simulink model "SWC_FDC_type"  (R2021b)
settings: Solver=FixedStepDiscrete  StartTime=0.0  StopTime=10.0  FixedStep=0.001  RelTol=1e-3
values from neighbouring files (symbols this model uses):
  DID_VCUKey = uint16(0x0202)    [vcu_local_hdr.m]
  DID_XWD = uint16(513)    [vcu_local_hdr.m]
  DIDLen_DKCKey = uint16(8)    [vcu_local_hdr.m]
  DIDLen_DynoMode = uint16(1)    [vcu_local_hdr.m]
  DIDLen_LFLowPresThre = uint16(1)    [vcu_local_hdr.m]
  DIDLen_LFSensorID = uint16(4)    [vcu_local_hdr.m]
  DIDLen_LRLowPresThre = uint16(1)    [vcu_local_hdr.m]
  DIDLen_LRSensorID = uint16(4)    [vcu_local_hdr.m]
  DIDLen_RFLowPresThre = uint16(1)    [vcu_local_hdr.m]
  DIDLen_RFSensorID = uint16(4)    [vcu_local_hdr.m]
  DIDLen_RRLowPresThre = uint16(1)    [vcu_local_hdr.m]
  DIDLen_RRSensorID = uint16(4)    [vcu_local_hdr.m]
  DIDLen_SensorMode = uint16(1)    [vcu_local_hdr.m]
  DIDLen_TPMSLearnSta = uint16(1)    [vcu_local_hdr.m]
  DIDLen_WhlPres = uint16(4)    [vcu_local_hdr.m]
  DIDLen_WhlSensorBattSta = uint16(1)    [vcu_local_hdr.m]
  DIDLen_WhlTmp = uint16(4)    [vcu_local_hdr.m]
  DIDLen_XWDMode = uint16(1)    [vcu_local_hdr.m]
  DIDNum_DKCKey = uint16(0x0202)    [vcu_local_hdr.m]
  DIDNum_DynoMode = uint16(0x0203)    [vcu_local_hdr.m]
  DIDNum_LFLowPresThre = uint16(0x0B08)    [vcu_local_hdr.m]
  DIDNum_LFSensorID = uint16(0x0B01)    [vcu_local_hdr.m]
  DIDNum_LRLowPresThre = uint16(0x0B0A)    [vcu_local_hdr.m]
  DIDNum_LRSensorID = uint16(0x0B03)    [vcu_local_hdr.m]
  DIDNum_RFLowPresThre = uint16(0x0B09)    [vcu_local_hdr.m]
  DIDNum_RFSensorID = uint16(0x0B02)    [vcu_local_hdr.m]
  DIDNum_RRLowPresThre = uint16(0x0B0B)    [vcu_local_hdr.m]
  DIDNum_RRSensorID = uint16(0x0B04)    [vcu_local_hdr.m]
  DIDNum_SensorMode = uint16(0x0B0C)    [vcu_local_hdr.m]
  DIDNum_TPMSLearnSta = uint16(0x0B0D)    [vcu_local_hdr.m]
  DIDNum_WhlPres = uint16(0x0B05)    [vcu_local_hdr.m]
  DIDNum_WhlSensorBattSta = uint16(0x0B07)    [vcu_local_hdr.m]
  DIDNum_WhlTmp = uint16(0x0B06)    [vcu_local_hdr.m]
  DIDNum_XWDMode = uint16(0x0201)    [vcu_local_hdr.m]
  DIDVCUKeyLength = uint16(8)    [vcu_local_hdr.m]
  ENUM_DRIVETRAIN_AWD = uint8(  2  )    [vcu_local_hdr.m]
  ENUM_DRIVETRAIN_FWD = uint8(  1  )    [vcu_local_hdr.m]
  ENUM_DRIVETRAIN_RWD = uint8(  0  )    [vcu_local_hdr.m]
  ENUM_TPMSLearnStatus_LEARNED = uint8(  1  )    [vcu_local_hdr.m]
  ENUM_TPMSLearnStatus_LEARNFAIL = uint8(  2  )    [vcu_local_hdr.m]
  ENUM_TPMSLearnStatus_NOTLEARN = uint8(  0  )    [vcu_local_hdr.m]
  ENUM_TPMSSTA_FAT = uint8(  8  )    [vcu_local_hdr.m]
  ENUM_TPMSSTA_LOWBATTERY = uint8(  2  )    [vcu_local_hdr.m]
  FALSE = boolean( 0 )    [vcu_local_hdr.m]
  ONE_INT = uint8(1)    [vcu_local_hdr.m]
  P_boolean = 0.0    [APPTypes.sldd]
  TRUE = boolean( 1 )    [vcu_local_hdr.m]
  ZERO_FLOAT = single(0)    [vcu_local_hdr.m]
  ZERO_INT = uint8(0)    [vcu_local_hdr.m]
undefined symbols (not defined in the file or in its folder): f32_ApsOutVehSpdSig, KHAL_DKCDecryptEnable_flg_ovrdflg, KHAL_DKCDecryptEnable_flg_ovrdval, KHAL_RandomNumberY1_enum, KHAL_RandomNumberY2_enum, KHAL_RandomNumberY_ovrdflg, KHAL_TPMSRESBUTT_flg_ovrdflg, KHAL_TPMSRESBUTT_flg_ovrdval, R_DIDWriteCDD_CSOP_DIDSet_DKCKey, R_DIDWriteCDD_CSOP_DIDSet_DynoMode, R_DIDWriteCDD_CSOP_DIDSet_LFLowPresThre, R_DIDWriteCDD_CSOP_DIDSet_LFSensorID, R_DIDWriteCDD_CSOP_DIDSet_LRLowPresThre, R_DIDWriteCDD_CSOP_DIDSet_LRSensorID, R_DIDWriteCDD_CSOP_DIDSet_RFLowPresThre, R_DIDWriteCDD_CSOP_DIDSet_RFSensorID, R_DIDWriteCDD_CSOP_DIDSet_RRLowPresThre, R_DIDWriteCDD_CSOP_DIDSet_RRSensorID, R_DIDWriteCDD_CSOP_DIDSet_SensorMode, R_DIDWriteCDD_CSOP_DIDSet_TPMSLearnSta, R_DIDWriteCDD_CSOP_DIDSet_WhlPres, R_DIDWriteCDD_CSOP_DIDSet_WhlSensorBattSta, R_DIDWriteCDD_CSOP_DIDSet_WhlTmp, R_DIDWriteCDD_CSOP_DIDSet_XWDMode, R_E2E_CAN3_VCU1_CSOP_Write_CAN3_VCU1, R_E2E_CAN4_VCU1_CSOP_Write_CAN4_VCU1, R_FDCCDD_Inner_CSOP_FDC_AppCallSleep, R_HALIN_IMU_CSOP_IMUSetSta, R_HALINCDD_CSOP_PAS_Handler, R_HALINCDD_CSOP_UDS_Main, R_HALOUT_APS_CSOP_ApsOutput, R_HALOUTCDD_CSOP_AppNmStateReq, R_HALOUTCDD_CSOP_IVIReset, R_HALOUTCDD_CSOP_SetAcoreRebootCmdACK, R_HALOUTCDD_CSOP_SetSysPwrStat, R_HALOUTCDD_CSOP_SleepRequest, R_NVMReadCDD_Inner_NVM_ReadOperation, R_NVMWriteCDD_Inner_NVM_WriteOperation, R_UDSCDD_CSOP_DdmRestartOperationCycle, R_WDGCDD_CSOP_Call_Watchdog, R_WDGCDD_CSOP_Call_WDG_AppEnd, R_WDGCDD_CSOP_Call_WDG_AppStart, u16_DIDLen_DKCKey, u16_DIDLen_DynoMode, u16_DIDLen_LFLowPresThre, u16_DIDLen_LFSensorID, u16_DIDLen_LRLowPresThre, u16_DIDLen_LRSensorID, u16_DIDLen_RFLowPresThre, u16_DIDLen_RFSensorID, u16_DIDLen_RRLowPresThre, u16_DIDLen_RRSensorID, u16_DIDLen_SensorMode, u16_DIDLen_TPMSLearnSta, u16_DIDLen_WhlPres, u16_DIDLen_WhlSensorBattSta, u16_DIDLen_WhlTmp, u16_DIDLen_XWDMode, u16_DIDNum_DKCKey, u16_DIDNum_DynoMode ... (+42)
libraries: simulink x215, FVT_lib x137, hcu_lib x12, hdlsllib x9, app x1, halin x1, halout x1, inp x1, outp x1
(part 4 of 11)

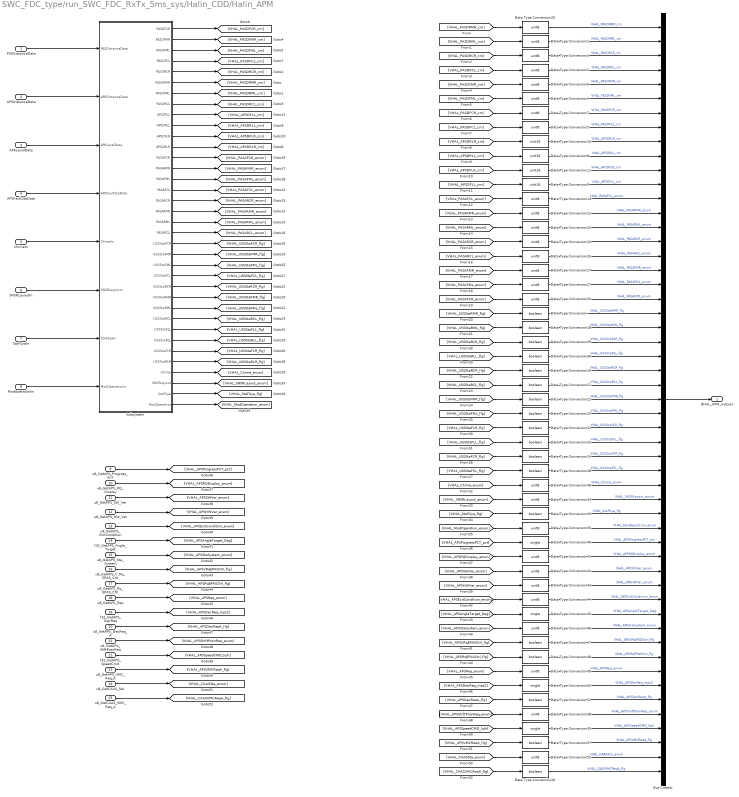
== system SWC_FDC_type/run_SWC_FDC_RxTx_5ms_sys/Halin_CDD/Halin_APM ==
  PASDistanceData : Inport
  APSDistanceData : Inport  Port=2
  APSLevelData : Inport  Port=3
  APSFaultStaData : Inport  Port=4
  ChimeIn : Inport  Port=5
  SNSRLayoutIn : Inport  Port=6
  StaFSyaIn : Inport  Port=7
  ModOperationIn : Inport  Port=8
  u8_GetAPS_Progress_PCT : Inport  Port=9
  u8_GetAPS_RQ_Display : Inport  Port=10
  u8_GetAPS_SW_Ver : Inport  Port=11
  u8_GetAPS_HW_Ver : Inport  Port=12
  u8_GetAPS_ExitCondition : Inport  Port=13
  f32_GetAPS_Angle_Target : Inport  Port=14
  u8_GetAPS_Sta_System : Inport  Port=15
  u8_GetAPS_V_Rq_EPAS_Ctrl : Inport  Port=16
  u8_GetAPS_Rq_EPAS_Ctrl : Inport  Port=17
  u8_GetAPS_Req : Inport  Port=18
  f32_GetAPS_DecReq : Inport  Port=19
  u8_GetAPS_DecReq_A : Inport  Port=20
  f32_GetAPS_SpeedCmd : Inport  Port=21
  u8_GetAPS_ShftPosnReq : Inport  Port=22
  u8_GetAPS_VMC_Req_A : Inport  Port=23
  u8_GetCAAS_Sta : Inport  Port=24
  u8_GetCAAS_VMC_Req_A : Inport  Port=25
  Bus Creator : BusCreator  Inputs=53
  Data Type Conversion{,16,18..19,21..24,28..33,37,47..48,51} (18 alike) : DataTypeConversion  OutDataTypeStr=boolean
  Data Type Conversion{1..7,12..15,17,20,25..27,34..36,38,41..44,46,49,52} (27 alike) : DataTypeConversion  OutDataTypeStr=uint8
  Data Type Conversion{8..11} (4 alike) : DataTypeConversion  OutDataTypeStr=uint16
  Data Type Conversion{39..40,45,50} (4 alike) : DataTypeConversion  OutDataTypeStr=single
  Subsystem : Subsystem
  BHAL_APM_outputs : Outport
  wires:
  [VHAL_USSStaRMR_flg] -> Data Type Conversion/1
  Data Type Conversion4/1 -> Bus Creator/6  "VHAL_PASDFML_cm"
  Subsystem/11(APSDFLR) -> [VHAL_APSDFLR_cm]
  [VHAL_PASARCL_enum] -> Data Type Conversion26/1
  Subsystem/36(ModOperation) -> [VHAL_ModOperation_enum]
  Bus Creator/1 -> BHAL_APM_outputs/1
  [VHAL_PASDRCR_cm] -> Data Type Conversion3/1
  [VHAL_PASDRML_cm] -> Data Type Conversion1/1
  Data Type Conversion15/1 -> Bus Creator/15  "VHAL_PASARML_enum"
  [VHAL_USSStaFCR_flg] -> Data Type Conversion24/1
  [VHAL_SNSRLayout_enum] -> Data Type Conversion34/1
  Subsystem/12(APSDRLR) -> [VHAL_APSDRLR_cm]
  Data Type Conversion3/1 -> Bus Creator/3  "VHAL_PASDRCR_cm"
  [VHAL_APSDRLR_cm] -> Data Type Conversion10/1
  Data Type Conversion12/1 -> Bus Creator/14  "VHAL_PASARMR_enum"
  Data Type Conversion33/1 -> Bus Creator/35  "VHAL_StaFSya_flg"
  [VHAL_PASARCR_enum] -> Data Type Conversion13/1
  Subsystem/9(APSDFLL) -> [VHAL_APSDFLL_cm]
  [VHAL_StaFSya_flg] -> Data Type Conversion33/1
  [VHAL_USSStaRLL_flg] -> Data Type Conversion30/1
  Subsystem/4(PASDFCL) -> [VHAL_PASDFCL_cm]
  Subsystem/35(StaFSya) -> [VHAL_StaFSya_flg]
  Subsystem/20(PASARCL) -> [VHAL_PASARCL_enum]
  [VHAL_PASDFML_cm] -> Data Type Conversion4/1
  [VHAL_PASDRMR_cm] -> Data Type Conversion20/1
  Subsystem/16(PASAFCL) -> [VHAL_PASAFCL_enum]
  [VHAL_USSStaFCL_flg] -> Data Type Conversion28/1
  Subsystem/18(PASARMR) -> [VHAL_PASARMR_enum]
  Data Type Conversion13/1 -> Bus Creator/16  "VHAL_PASARCR_enum"
  [VHAL_PASARML_enum] -> Data Type Conversion15/1
  [VHAL_APSDFLL_cm] -> Data Type Conversion9/1
  Subsystem/15(PASAFML) -> [VHAL_PASAFML_enum]
  [VHAL_USSStaFLL_flg] -> Data Type Conversion32/1
  Subsystem/8(PASDRCL) -> [VHAL_PASDRCL_cm]
  Subsystem/27(USSStaRML) -> [VHAL_USSStaRML_flg]
  Data Type Conversion6/1 -> Bus Creator/5  "VHAL_PASDFMR_cm"
  [VHAL_PASAFMR_enum] -> Data Type Conversion17/1
  Data Type Conversion28/1 -> Bus Creator/32  "VHAL_USSStaFCL_flg"
  Subsystem/3(PASDFML) -> [VHAL_PASDFML_cm]
  Data Type Conversion9/1 -> Bus Creator/12  "VHAL_APSDFLL_cm"
  Subsystem/24(USSStaFCL) -> [VHAL_USSStaFCL_flg]
  [VHAL_PASAFCL_enum] -> Data Type Conversion14/1
  [VHAL_USSStaFLR_flg] -> Data Type Conversion31/1
  Subsystem/34(SNSRLayout) -> [VHAL_SNSRLayout_enum]
  Subsystem/29(USSStaFLL) -> [VHAL_USSStaFLL_flg]
  Subsystem/21(USSStaFCR) -> [VHAL_USSStaFCR_flg]
  [VHAL_PASDRCL_cm] -> Data Type Conversion2/1
  Data Type Conversion14/1 -> Bus Creator/13  "VHAL_PASAFCL_enum"
  Subsystem/1(PASDFCR) -> [VHAL_PASDFCR_cm]
  Data Type Conversion7/1 -> Bus Creator/7  "VHAL_PASDFCR_cm"
  Subsystem/2(PASDFMR) -> [VHAL_PASDFMR_cm]
  Subsystem/30(USSStaRLL) -> [VHAL_USSStaRLL_flg]
  Data Type Conversion17/1 -> Bus Creator/18  "VHAL_PASAFMR_enum"
  [VHAL_PASARMR_enum] -> Data Type Conversion12/1
  Data Type Conversion32/1 -> Bus Creator/30  "VHAL_USSStaFLL_flg"
  Subsystem/7(PASDRML) -> [VHAL_PASDRML_cm]
  Subsystem/26(USSStaRMR) -> [VHAL_USSStaRMR_flg]
  Data Type Conversion20/1 -> Bus Creator/1  "VHAL_PASDRMR_cm"
  [VHAL_USSStaRCL_flg] -> Data Type Conversion21/1
  Subsystem/10(APSDRLL) -> [VHAL_APSDRLL_cm]
  Data Type Conversion34/1 -> Bus Creator/34  "VHAL_SNSRLayout_enum"
  [VHAL_Chime_enum] -> Data Type Conversion36/1
  Data Type Conversion18/1 -> Bus Creator/22  "VHAL_USSStaRML_flg"
  [VHAL_PASDFMR_cm] -> Data Type Conversion6/1
  Data Type Conversion31/1 -> Bus Creator/29  "VHAL_USSStaFLR_flg"
  Data Type Conversion10/1 -> Bus Creator/9  "VHAL_APSDRLR_cm"
  Data Type Conversion35/1 -> Bus Creator/36  "VHAL_ModOperation_enum"
  Subsystem/31(USSStaFLR) -> [VHAL_USSStaFLR_flg]
  Data Type Conversion8/1 -> Bus Creator/10  "VHAL_APSDRLL_cm"
  [VHAL_USSStaRML_flg] -> Data Type Conversion18/1
  Subsystem/19(PASARML) -> [VHAL_PASARML_enum]
  [VHAL_USSStaFMR_flg] -> Data Type Conversion22/1
  Subsystem/22(USSStaFMR) -> [VHAL_USSStaFMR_flg]
  Data Type Conversion25/1 -> Bus Creator/20  "VHAL_PASAFCR_enum"
  Subsystem/33(Chime) -> [VHAL_Chime_enum]
  Data Type Conversion11/1 -> Bus Creator/11  "VHAL_APSDFLR_cm"
  Data Type Conversion36/1 -> Bus Creator/33  "VHAL_Chime_enum"
  [VHAL_APSDFLR_cm] -> Data Type Conversion11/1
  Subsystem/13(PASAFCR) -> [VHAL_PASAFCR_enum]
  [VHAL_PASDFCL_cm] -> Data Type Conversion5/1
  Data Type Conversion/1 -> Bus Creator/21  "VHAL_USSStaRMR_flg"
  Data Type Conversion2/1 -> Bus Creator/4  "VHAL_PASDRCL_cm"
  [VHAL_USSStaFML_flg] -> Data Type Conversion23/1
  Data Type Conversion1/1 -> Bus Creator/2  "VHAL_PASDRML_cm"
  [VHAL_USSStaRCR_flg] -> Data Type Conversion19/1
  Subsystem/25(USSStaRCR) -> [VHAL_USSStaRCR_flg]
  Subsystem/28(USSStaRCL) -> [VHAL_USSStaRCL_flg]
  [VHAL_ModOperation_enum] -> Data Type Conversion35/1
  Data Type Conversion19/1 -> Bus Creator/25  "VHAL_USSStaRCR_flg"
  Subsystem/5(PASDRCR) -> [VHAL_PASDRCR_cm]
  Data Type Conversion26/1 -> Bus Creator/17  "VHAL_PASARCL_enum"
  Data Type Conversion27/1 -> Bus Creator/19  "VHAL_PASAFML_enum"
  Subsystem/23(USSStaFML) -> [VHAL_USSStaFML_flg]
  Subsystem/17(PASARCR) -> [VHAL_PASARCR_enum]
  [VHAL_APSDRLL_cm] -> Data Type Conversion8/1
  Subsystem/6(PASDRMR) -> [VHAL_PASDRMR_cm]
  Data Type Conversion21/1 -> Bus Creator/26  "VHAL_USSStaRCL_flg"
  Data Type Conversion24/1 -> Bus Creator/31  "VHAL_USSStaFCR_flg"
  Data Type Conversion23/1 -> Bus Creator/28  "VHAL_USSStaFML_flg"
  Data Type Conversion5/1 -> Bus Creator/8  "VHAL_PASDFCL_cm"
  [VHAL_PASAFCR_enum] -> Data Type Conversion25/1
  [VHAL_PASDFCR_cm] -> Data Type Conversion7/1
  Data Type Conversion29/1 -> Bus Creator/23  "VHAL_USSStaRLR_flg"
  [VHAL_USSStaRLR_flg] -> Data Type Conversion29/1
  Subsystem/14(PASAFMR) -> [VHAL_PASAFMR_enum]
  Data Type Conversion30/1 -> Bus Creator/24  "VHAL_USSStaRLL_flg"
  Subsystem/32(USSStaRLR) -> [VHAL_USSStaRLR_flg]
  [VHAL_PASAFML_enum] -> Data Type Conversion27/1
  Data Type Conversion22/1 -> Bus Creator/27  "VHAL_USSStaFMR_flg"
  APSDistanceData/1 -> Subsystem/2(APSDistanceData)
  APSFaultStaData/1 -> Subsystem/4(APSFaultStaData)
  APSLevelData/1 -> Subsystem/3(APSLevelData)
  ChimeIn/1 -> Subsystem/5(ChimeIn)
  SNSRLayoutIn/1 -> Subsystem/6(SNSRLayoutIn)
  StaFSyaIn/1 -> Subsystem/7(StaFSyaIn)
  ModOperationIn/1 -> Subsystem/8(ModOperationIn)
  PASDistanceData/1 -> Subsystem/1(PASDistanceData)
  u8_GetAPS_HW_Ver/1 -> [VHAL_APSHWVer_enum]
  u8_GetAPS_Progress_PCT/1 -> [VHAL_APSProgressPCT_pct]
  u8_GetAPS_Req/1 -> [VHAL_APSReq_enum]
  u8_GetAPS_Sta_System/1 -> [VHAL_APSStaSystem_enum]
  u8_GetAPS_SW_Ver/1 -> [VHAL_APSSWVer_enum]
  u8_GetAPS_V_Rq_EPAS_Ctrl/1 -> [VHAL_APSVRqEPASCtrl_flg]
  u8_GetAPS_ExitCondition/1 -> [VHAL_APSExitCondition_enum]
  u8_GetCAAS_Sta/1 -> [VHAL_CAASSta_enum]
  u8_GetAPS_VMC_Req_A/1 -> [VHAL_APSVMCReqA_flg]
  f32_GetAPS_SpeedCmd/1 -> [VHAL_APSSpeedCMD_kph]
  u8_GetAPS_Rq_EPAS_Ctrl/1 -> [VHAL_APSRqEPASCtrl_flg]
  u8_GetAPS_ShftPosnReq/1 -> [VHAL_APSShiftPosnReq_enum]
  u8_GetAPS_DecReq_A/1 -> [VHAL_APSDecReqA_flg]
  f32_GetAPS_Angle_Target/1 -> [VHAL_APSAngleTarget_Deg]
  u8_GetAPS_RQ_Display/1 -> [VHAL_APSRQDisplay_enum]
  f32_GetAPS_DecReq/1 -> [VHAL_APSDecReq_mps2]
  u8_GetCAAS_VMC_Req_A/1 -> [VHAL_CAASVMCReqA_flg]
  Data Type Conversion47/1 -> Bus Creator/44  "VHAL_APSVRqEPASCtrl_flg"
  Data Type Conversion50/1 -> Bus Creator/47  "VHAL_APSDecReq_mps2"
  Data Type Conversion39/1 -> Bus Creator/50  "VHAL_APSSpeedCMD_kph"
  Data Type Conversion43/1 -> Bus Creator/40  "VHAL_APSHWVer_enum"
  Data Type Conversion38/1 -> Bus Creator/49  "VHAL_APSShiftPosnReq_enum"
  Data Type Conversion42/1 -> Bus Creator/39  "VHAL_APSSWVer_enum"
  [VHAL_APSVRqEPASCtrl_flg] -> Data Type Conversion47/1
  Data Type Conversion51/1 -> Bus Creator/48  "VHAL_APSDecReqA_flg"
  Data Type Conversion46/1 -> Bus Creator/43  "VHAL_APSStaSystem_enum"
  Data Type Conversion44/1 -> Bus Creator/41  "VHAL_APSExitCondition_enum"
  [VHAL_APSVMCReqA_flg] -> Data Type Conversion37/1
  [VHAL_APSReq_enum] -> Data Type Conversion49/1
  [VHAL_APSSpeedCMD_kph] -> Data Type Conversion39/1
  Data Type Conversion48/1 -> Bus Creator/45  "VHAL_APSRqEPASCtrl_flg"
  [VHAL_APSShiftPosnReq_enum] -> Data Type Conversion38/1
  Data Type Conversion52/1 -> Bus Creator/52  "VHAL_CAASSta_enum"
  Data Type Conversion45/1 -> Bus Creator/42  "VHAL_APSAngleTarget_Deg"
  Data Type Conversion49/1 -> Bus Creator/46  "VHAL_APSReq_enum"
  [VHAL_CAASSta_enum] -> Data Type Conversion52/1
  [VHAL_APSRqEPASCtrl_flg] -> Data Type Conversion48/1
  [VHAL_APSStaSystem_enum] -> Data Type Conversion46/1
  Data Type Conversion40/1 -> Bus Creator/37  "VHAL_APSProgressPCT_pct"
  [VHAL_APSExitCondition_enum] -> Data Type Conversion44/1
  [VHAL_APSSWVer_enum] -> Data Type Conversion42/1
  [VHAL_APSHWVer_enum] -> Data Type Conversion43/1
  [VHAL_APSAngleTarget_Deg] -> Data Type Conversion45/1
  [VHAL_APSDecReq_mps2] -> Data Type Conversion50/1
  [VHAL_APSProgressPCT_pct] -> Data Type Conversion40/1
  [VHAL_APSDecReqA_flg] -> Data Type Conversion51/1
  [VHAL_APSRQDisplay_enum] -> Data Type Conversion41/1
  Data Type Conversion41/1 -> Bus Creator/38  "VHAL_APSRQDisplay_enum"
  Data Type Conversion37/1 -> Bus Creator/51  "VHAL_APSVMCReqA_flg"
  [VHAL_CAASVMCReqA_flg] -> Data Type Conversion16/1
  Data Type Conversion16/1 -> Bus Creator/53  "VHAL_CAASVMCReqA_flg"

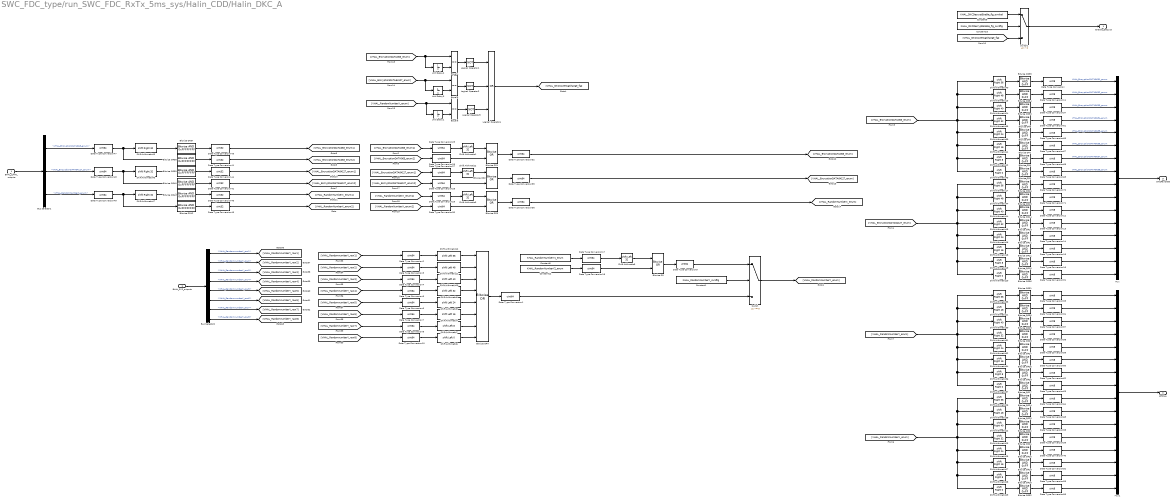
== system SWC_FDC_type/run_SWC_FDC_RxTx_5ms_sys/Halin_CDD/Halin_DKC_A ==
  BHAL_CAN4_outputs : Inport
  BHAL_SYS_outputs : Inport  Port=2
  Bitwise OR{,1..3} (4 alike) : simulink/Logic and Bit Operations/Bitwise Operator  logicop=OR  UseBitMask=off  NumInputPorts=2  BitMask=bin2dec('11011001')  BitMaskRealWorld=Stored Integer
  Bitwise OR{5..36} (32 alike) : simulink/Logic and Bit Operations/Bitwise Operator  logicop=AND  UseBitMask=on  BitMask=0xFF  BitMaskRealWorld=Stored Integer
  Bitwise OR{37..42} (6 alike) : simulink/Logic and Bit Operations/Bitwise Operator  logicop=AND  UseBitMask=on  BitMask=0xFFFFFFFF  BitMaskRealWorld=Stored Integer
  Bitwise OR4 : simulink/Logic and Bit Operations/Bitwise Operator  logicop=OR  UseBitMask=off  NumInputPorts=8  BitMask=bin2dec('11011001')  BitMaskRealWorld=Stored Integer
  Bus Selector1 : BusSelector  OutputSignals=VHAL_EncryptionDATA063_enum,VHAL_EncryptionDATA64127_enum,VHAL_RandomNumberX_enum
  Bus Selector2 : BusSelector  OutputSignals=VHAL_RandomnumberY_raw1,VHAL_RandomnumberY_raw2,VHAL_RandomnumberY_raw3,VHAL_RandomnumberY_raw4,VHAL_RandomnumberY_raw5,VHAL_RandomnumberY_raw6,VHAL_RandomnumberY_raw7,VHAL_RandomnumberY_raw8
  Constant1 : Constant  Value=KHAL_RandomNumberY_ovrdflg  OutDataTypeStr=uint64
  Constant10 : Constant  Value=KHAL_DKCDecryptEnable_flg_ovrdflg
  Constant12 : Constant  Value=KHAL_RandomNumberY2_enum  OutDataTypeStr=uint64
  Constant5 : Constant  Value=KHAL_RandomNumberY1_enum  OutDataTypeStr=uint64
  Constant9 : Constant  Value=KHAL_DKCDecryptEnable_flg_ovrdval
  Data Type Conversion{,11..16,31,33..34,37..40,52,55..71} (32 alike) : DataTypeConversion  OutDataTypeStr=uint8
  Data Type Conversion{1..10,17..18,25..30,32,35..36,47..49} (24 alike) : DataTypeConversion  OutDataTypeStr=uint64
  Data Type Conversion{41..46} (6 alike) : DataTypeConversion  OutDataTypeStr=uint32
  Equal4 : RelationalOperator  Operator===  OutDataTypeStr=boolean  RndMeth=Simplest
  Equal5 : RelationalOperator  Operator===  OutDataTypeStr=boolean  RndMeth=Simplest
  Equal6 : RelationalOperator  Operator===  OutDataTypeStr=boolean  RndMeth=Simplest
  Logical Operator1 : Logic  Operator=NOT  AllPortsSameDT=off  OutDataTypeStr=boolean
  Logical Operator2 : Logic  Operator=NOT  AllPortsSameDT=off  OutDataTypeStr=boolean
  Logical Operator3 : Logic  Operator=NOT  AllPortsSameDT=off  OutDataTypeStr=boolean
  Logical Operator4 : Logic  Operator=OR  Inputs=3  AllPortsSameDT=off  OutDataTypeStr=boolean
  Mux : Mux  Inputs=16
  Mux1 : Mux  Inputs=16
  Shift Arithmetic{1..3,5,9} (5 alike) : ArithShift  BitShiftNumber=32  BitShiftDirection=Left
  Shift Arithmetic10 : ArithShift  BitShiftNumber=40  BitShiftDirection=Left
  Shift Arithmetic11 : ArithShift  BitShiftNumber=48  BitShiftDirection=Left
  Shift Arithmetic12 : ArithShift  BitShiftNumber=56  BitShiftDirection=Left
  Shift Arithmetic{13,21,38,44} (4 alike) : ArithShift  BitShiftNumber=48  BitShiftDirection=Right
  Shift Arithmetic{14,22,24,30} (4 alike) : ArithShift  BitShiftNumber=40  BitShiftDirection=Right
  Shift Arithmetic{15,23,31,35,45..47} (7 alike) : ArithShift  BitShiftNumber=32  BitShiftDirection=Right
  Shift Arithmetic{16,25,32,39} (4 alike) : ArithShift  BitShiftNumber=24  BitShiftDirection=Right
  Shift Arithmetic{17,26,33,40} (4 alike) : ArithShift  BitShiftNumber=56  BitShiftDirection=Right
  Shift Arithmetic{18,27,34,41} (4 alike) : ArithShift  BitShiftNumber=16  BitShiftDirection=Right
  Shift Arithmetic{19,28,36,42} (4 alike) : ArithShift  BitShiftNumber=8  BitShiftDirection=Right
  Shift Arithmetic{20,29,37,43} (4 alike) : ArithShift  BitShiftDirection=Right
  Shift Arithmetic4 : ArithShift  BitShiftNumber=16  BitShiftDirection=Left
  Shift Arithmetic6 : ArithShift  BitShiftDirection=Left
  Shift Arithmetic7 : ArithShift  BitShiftNumber=8  BitShiftDirection=Left
  Shift Arithmetic8 : ArithShift  BitShiftNumber=24  BitShiftDirection=Left
  Switch : Switch  Criteria=u2 ~= 0
  Switch1 : Switch  Criteria=u2 > Threshold
  Unit Delay1 : UnitDelay  SampleTime=-1  HasFrameUpgradeWarning=on
  Unit Delay2 : UnitDelay  SampleTime=-1  HasFrameUpgradeWarning=on
  Unit Delay3 : UnitDelay  SampleTime=-1  HasFrameUpgradeWarning=on
  Enable_Decrypt : Outport
  AESKey : Outport  Port=2
  DKCRawData : Outport  Port=3
  wires:
  Data Type Conversion8/1 -> Shift Arithmetic7/1
  Bitwise OR5/1 -> Data Type Conversion69/1
  [VHAL_RandomNumberX_enum] -> Shift Arithmetic38/1, Shift Arithmetic26/1, Shift Arithmetic22/1, Shift Arithmetic25/1, Shift Arithmetic27/1, Shift Arithmetic29/1, Shift Arithmetic28/1, Shift Arithmetic23/1
  Shift Arithmetic17/1 -> Bitwise OR16/1
  Data Type Conversion52/1 -> Mux1/14
  Bitwise OR35/1 -> Data Type Conversion/1
  Shift Arithmetic13/1 -> Bitwise OR34/1
  Data Type Conversion42/1 -> [VHAL_EncryptionDATA64127_enum2]
  Bitwise OR/1 -> Data Type Conversion9/1
  [VHAL_EncryptionDATA64127_enum] -> Shift Arithmetic15/1, Shift Arithmetic19/1, Shift Arithmetic20/1, Shift Arithmetic18/1, Shift Arithmetic16/1, Shift Arithmetic14/1, Shift Arithmetic17/1, Shift Arithmetic44/1
  [VHAL_RandomnumberY_raw5] -> Data Type Conversion6/1
  Shift Arithmetic7/1 -> Bitwise OR4/7
  [VHAL_RandomnumberY_raw4] -> Data Type Conversion5/1
  [VHAL_RandomNumberX_enum] -> Equal6/1, Unit Delay1/1
  [VHAL_EncryptionDATA063_enum] -> Shift Arithmetic13/1, Shift Arithmetic40/1, Shift Arithmetic24/1, Shift Arithmetic39/1, Shift Arithmetic41/1, Shift Arithmetic43/1, Shift Arithmetic42/1, Shift Arithmetic35/1
  Bus Selector2/3 -> [VHAL_RandomnumberY_raw3]  "<VHAL_RandomnumberY_raw3>"
  Bitwise OR15/1 -> Data Type Conversion71/1
  Bus Selector2/2 -> [VHAL_RandomnumberY_raw2]  "<VHAL_RandomnumberY_raw2>"
  [VHAL_RandomnumberY_raw1] -> Data Type Conversion2/1
  Data Type Conversion69/1 -> Mux/8  "VHAL_EncryptionDATA0638_enum"
  Data Type Conversion37/1 -> Mux/3  "VHAL_EncryptionDATA0633_enum"
  Data Type Conversion5/1 -> Shift Arithmetic9/1
  Bitwise OR8/1 -> Data Type Conversion66/1
  Bitwise OR14/1 -> Data Type Conversion12/1
  Bus Selector2/1 -> [VHAL_RandomnumberY_raw1]  "<VHAL_RandomnumberY_raw1>"
  Bitwise OR17/1 -> Data Type Conversion63/1
  Data Type Conversion34/1 -> Mux1/2
  Bus Selector2/5 -> [VHAL_RandomnumberY_raw5]  "<VHAL_RandomnumberY_raw5>"
  Shift Arithmetic35/1 -> Bitwise OR9/1
  Data Type Conversion67/1 -> Mux/6  "VHAL_EncryptionDATA0636_enum"
  Bus Selector2/6 -> [VHAL_RandomnumberY_raw6]  "<VHAL_RandomnumberY_raw6>"
  Data Type Conversion9/1 -> Switch/1
  Data Type Conversion10/1 -> Shift Arithmetic6/1
  Data Type Conversion45/1 -> [VHAL_RandomNumberX_enum2]
  Data Type Conversion13/1 -> Mux/12
  Data Type Conversion1/1 -> Switch/3
  [VHAL_RandomnumberY_raw2] -> Data Type Conversion3/1
  BHAL_SYS_outputs/1 -> Bus Selector2/1
  Shift Arithmetic25/1 -> Bitwise OR20/1
  [VHAL_EncryptionDATA063_enum1] -> Data Type Conversion25/1
  Logical Operator3/1 -> Logical Operator4/3
  Shift Arithmetic6/1 -> Bitwise OR4/8
  Data Type Conversion70/1 -> Mux/9
  Data Type Conversion66/1 -> Mux/5  "VHAL_EncryptionDATA0635_enum"
  [VHAL_EncryptionDATA64127_enum] -> Equal5/1, Unit Delay3/1
  Data Type Conversion14/1 -> Mux/13
  Shift Arithmetic10/1 -> Bitwise OR4/3
  Data Type Conversion40/1 -> Mux1/13
  Unit Delay1/1 -> Equal6/2
  Data Type Conversion43/1 -> [VHAL_EncryptionDATA063_enum1]
  Unit Delay3/1 -> Equal5/2
  Bitwise OR31/1 -> Data Type Conversion33/1
  Shift Arithmetic12/1 -> Bitwise OR4/1
  [VHAL_RandomnumberY_raw3] -> Data Type Conversion4/1
  Shift Arithmetic28/1 -> Bitwise OR18/1
  Constant1/1 -> Switch/2
  Data Type Conversion7/1 -> Shift Arithmetic4/1
  Bitwise OR4/1 -> Data Type Conversion1/1
  Bitwise OR21/1 -> Data Type Conversion39/1
  Shift Arithmetic11/1 -> Bitwise OR4/2
  Data Type Conversion31/1 -> Mux/16
  Shift Arithmetic2/1 -> Bitwise OR2/1
  Data Type Conversion68/1 -> Mux/7  "VHAL_EncryptionDATA0637_enum"
  Data Type Conversion4/1 -> Shift Arithmetic10/1
  Bus Selector2/7 -> [VHAL_RandomnumberY_raw7]  "<VHAL_RandomnumberY_raw7>"
  Data Type Conversion12/1 -> Mux/11
  Data Type Conversion30/1 -> Bitwise OR3/2
  Data Type Conversion32/1 -> [VHAL_EncryptionDATA063_enum]
  [VHAL_RandomNumberY_enum] -> Shift Arithmetic31/1, Shift Arithmetic36/1, Shift Arithmetic37/1, Shift Arithmetic34/1, Shift Arithmetic32/1, Shift Arithmetic30/1, Shift Arithmetic33/1, Shift Arithmetic21/1
  Shift Arithmetic14/1 -> Bitwise OR14/1
  Data Type Conversion55/1 -> Mux1/15
  Shift Arithmetic33/1 -> Bitwise OR31/1
  Data Type Conversion59/1 -> Mux1/5
  Shift Arithmetic21/1 -> Bitwise OR30/1
  Shift Arithmetic18/1 -> Bitwise OR11/1
  [VHAL_EncryptionDATA64127_enum2] -> Data Type Conversion28/1
  [VHAL_RandomNumberX_enum2] -> Data Type Conversion30/1
  Shift Arithmetic1/1 -> Bitwise OR1/1
  Data Type Conversion18/1 -> Bitwise OR/2
  Shift Arithmetic26/1 -> Bitwise OR24/1
  Shift Arithmetic15/1 -> Bitwise OR13/1
  Shift Arithmetic23/1 -> Bitwise OR21/1
  Data Type Conversion39/1 -> Mux1/12
  Bitwise OR2/1 -> Data Type Conversion35/1
  Bitwise OR25/1 -> Data Type Conversion62/1
  Bitwise OR36/1 -> Data Type Conversion31/1
  Data Type Conversion15/1 -> Mux/14
  Bitwise OR11/1 -> Data Type Conversion15/1
  Switch/1 -> [VHAL_RandomNumberY_enum]
  Shift Arithmetic9/1 -> Bitwise OR4/4
  Bitwise OR7/1 -> Data Type Conversion67/1
  Data Type Conversion35/1 -> [VHAL_EncryptionDATA64127_enum]
  Shift Arithmetic29/1 -> Bitwise OR32/1
  Data Type Conversion58/1 -> Mux1/4
  Bitwise OR1/1 -> Data Type Conversion32/1
  Bitwise OR27/1 -> Data Type Conversion59/1
  Data Type Conversion33/1 -> Mux1/1
  Bitwise OR24/1 -> Data Type Conversion64/1
  Bitwise OR22/1 -> Data Type Conversion38/1
  Data Type Conversion/1 -> Mux/1  "VHAL_EncryptionDATA0631_enum"
  Equal5/1 -> Logical Operator2/1
  [VHAL_EncryptionDATA063_enum2] -> Data Type Conversion26/1
  [VHAL_RandomnumberY_raw8] -> Data Type Conversion10/1
  [VHAL_EncryptionDATA063_enum] -> Equal4/1, Unit Delay2/1
  Data Type Conversion36/1 -> [VHAL_RandomNumberX_enum]
  Data Type Conversion29/1 -> Shift Arithmetic3/1
  Shift Arithmetic8/1 -> Bitwise OR4/5
  Bitwise OR29/1 -> Data Type Conversion57/1
  Data Type Conversion28/1 -> Bitwise OR2/2
  Constant12/1 -> Data Type Conversion18/1
  Data Type Conversion26/1 -> Bitwise OR1/2
  Shift Arithmetic31/1 -> Bitwise OR28/1
  Data Type Conversion25/1 -> Shift Arithmetic1/1
  Logical Operator2/1 -> Logical Operator4/2
  [VHAL_RandomNumberX_enum1] -> Data Type Conversion29/1
  Constant5/1 -> Data Type Conversion17/1
  Bitwise OR23/1 -> Data Type Conversion65/1
  Shift Arithmetic4/1 -> Bitwise OR4/6
  Data Type Conversion41/1 -> [VHAL_EncryptionDATA063_enum2]
  Data Type Conversion2/1 -> Shift Arithmetic12/1
  Shift Arithmetic24/1 -> Bitwise OR33/1
  Shift Arithmetic3/1 -> Bitwise OR3/1
  [VHAL_RandomnumberY_raw7] -> Data Type Conversion8/1
  Bus Selector2/8 -> [VHAL_RandomnumberY_raw8]  "<VHAL_RandomnumberY_raw8>"
  Shift Arithmetic41/1 -> Bitwise OR7/1
  [VHAL_EncryptionDATA64127_enum1] -> Data Type Conversion27/1
  [VHAL_RandomnumberY_raw6] -> Data Type Conversion7/1
  Bitwise OR3/1 -> Data Type Conversion36/1
  Data Type Conversion17/1 -> Shift Arithmetic5/1
  Logical Operator4/1 -> [VHAL_DKCCANMsgChange_flg]
  Data Type Conversion44/1 -> [VHAL_EncryptionDATA64127_enum1]
  Data Type Conversion11/1 -> Mux/2  "VHAL_EncryptionDATA0632_enum"
  Data Type Conversion3/1 -> Shift Arithmetic11/1
  Shift Arithmetic36/1 -> Bitwise OR25/1
  Data Type Conversion27/1 -> Shift Arithmetic2/1
  Unit Delay2/1 -> Equal4/2
  Equal6/1 -> Logical Operator3/1
  Bus Selector2/4 -> [VHAL_RandomnumberY_raw4]  "<VHAL_RandomnumberY_raw4>"
  Shift Arithmetic5/1 -> Bitwise OR/1
  Data Type Conversion6/1 -> Shift Arithmetic8/1
  Equal4/1 -> Logical Operator1/1
  Data Type Conversion46/1 -> [VHAL_RandomNumberX_enum1]
  Data Type Conversion71/1 -> Mux/10
  Logical Operator1/1 -> Logical Operator4/1
  Shift Arithmetic44/1 -> Bitwise OR15/1
  Shift Arithmetic43/1 -> Bitwise OR5/1
  Shift Arithmetic27/1 -> Bitwise OR19/1
  Shift Arithmetic34/1 -> Bitwise OR26/1
  Bitwise OR9/1 -> Data Type Conversion61/1
  Data Type Conversion62/1 -> Mux1/7
  Shift Arithmetic16/1 -> Bitwise OR12/1
  Shift Arithmetic19/1 -> Bitwise OR10/1
  Mux/1 -> DKCRawData/1
  Bitwise OR6/1 -> Data Type Conversion68/1
  Shift Arithmetic40/1 -> Bitwise OR35/1
  Bitwise OR26/1 -> Data Type Conversion60/1
  Bitwise OR12/1 -> Data Type Conversion14/1
  Data Type Conversion63/1 -> Mux1/8
  Data Type Conversion65/1 -> Mux1/10
  Shift Arithmetic42/1 -> Bitwise OR6/1
  Bitwise OR16/1 -> Data Type Conversion70/1
  Bitwise OR33/1 -> Data Type Conversion37/1
  Shift Arithmetic22/1 -> Bitwise OR22/1
  Bitwise OR32/1 -> Data Type Conversion56/1
  Data Type Conversion38/1 -> Mux1/11
  Shift Arithmetic39/1 -> Bitwise OR8/1
  Bitwise OR10/1 -> Data Type Conversion16/1
  Data Type Conversion16/1 -> Mux/15
  Data Type Conversion56/1 -> Mux1/16
  Shift Arithmetic20/1 -> Bitwise OR36/1
  Bitwise OR13/1 -> Data Type Conversion13/1
  Bitwise OR19/1 -> Data Type Conversion52/1
  Bitwise OR18/1 -> Data Type Conversion55/1
  Data Type Conversion64/1 -> Mux1/9
  Data Type Conversion61/1 -> Mux/4  "VHAL_EncryptionDATA0634_enum"
  Shift Arithmetic32/1 -> Bitwise OR27/1
  Data Type Conversion60/1 -> Mux1/6
  Bitwise OR28/1 -> Data Type Conversion58/1
  Shift Arithmetic38/1 -> Bitwise OR23/1
  Bitwise OR20/1 -> Data Type Conversion40/1
  Shift Arithmetic30/1 -> Bitwise OR29/1
  Bitwise OR34/1 -> Data Type Conversion11/1
  Shift Arithmetic37/1 -> Bitwise OR17/1
  Data Type Conversion57/1 -> Mux1/3
  Bitwise OR30/1 -> Data Type Conversion34/1
  Mux1/1 -> AESKey/1
  Constant9/1 -> Switch1/1
  [VHAL_DKCCANMsgChange_flg] -> Switch1/3
  Constant10/1 -> Switch1/2
  Switch1/1 -> Enable_Decrypt/1
  Bitwise OR42/1 -> Data Type Conversion45/1
  Bitwise OR40/1 -> Data Type Conversion42/1
  Bus Selector1/1 -> Data Type Conversion47/1  "<VHAL_EncryptionDATA063_enum>"
  Shift Arithmetic46/1 -> Bitwise OR39/1
  Bitwise OR38/1 -> Data Type Conversion41/1
  Data Type Conversion49/1 -> Bitwise OR42/1, Shift Arithmetic47/1
  Bitwise OR41/1 -> Data Type Conversion46/1
  Data Type Conversion48/1 -> Bitwise OR40/1, Shift Arithmetic46/1
  Shift Arithmetic47/1 -> Bitwise OR41/1
  Shift Arithmetic45/1 -> Bitwise OR37/1
  Data Type Conversion47/1 -> Bitwise OR38/1, Shift Arithmetic45/1
  Bus Selector1/2 -> Data Type Conversion48/1  "<VHAL_EncryptionDATA64127_enum>"
  Bitwise OR39/1 -> Data Type Conversion44/1
  Bitwise OR37/1 -> Data Type Conversion43/1
  Bus Selector1/3 -> Data Type Conversion49/1  "<VHAL_RandomNumberX_enum>"
  BHAL_CAN4_outputs/1 -> Bus Selector1/1

== system SWC_FDC_type/run_SWC_FDC_RxTx_5ms_sys/Halin_CDD/Halin_GPIO ==
  VHAL_AccelPedal1Vol_Raw : Inport
  VHAL_AccelPedal2Vol_Raw : Inport  Port=2
  VHAL_BrakeSWGPIO_flg : Inport  Port=3
  VHAL_HoodSW_flg : Inport  Port=4
  VHAL_TailgateSW_flg : Inport  Port=5
  VHAL_DrDoorSW_flg : Inport  Port=6
  VHAL_PsDoorSW_flg : Inport  Port=7
  VHAL_RRDoorSW_flg : Inport  Port=8
  VHAL_RLDoorSW_flg : Inport  Port=9
  VHAL_CentralDoorLockSW_flg : Inport  Port=10
  VHAL_HazardSW_flg : Inport  Port=11
  VHAL_BrakeLampSW_flg : Inport  Port=12
  VHAL_TrunkHanSW_flg : Inport  Port=13
  VHAL_SeatSW_flg : Inport  Port=14
  VHAL_CrashSignalGPIO_flg : Inport  Port=15
  u8_HWID_4byte : Inport  Port=16
  Bus Creator : BusCreator  Inputs=21
  Data Type Conversion{1,3..4,17} (4 alike) : DataTypeConversion  OutDataTypeStr=single
  Data Type Conversion{2,5..10,12..16,18} (13 alike) : DataTypeConversion  OutDataTypeStr=boolean
  Data Type Conversion{11,19..21} (4 alike) : DataTypeConversion  OutDataTypeStr=uint8
  Demux : Demux
  Gain : Gain  Gain=5/4095
  Gain1 : Gain  Gain=5/4095
  Ground3 : Ground
  Ground4 : Ground
  Logical Operator{2..13} (12 alike) : Logic  Operator=NOT  AllPortsSameDT=off  OutDataTypeStr=boolean
  BHAL_GPIO_outputs : Outport
  wires:
  Data Type Conversion7/1 -> Bus Creator/7  "VHAL_TailgateSW_flg"
  Data Type Conversion9/1 -> Bus Creator/9  "VHAL_PsDoorSW_flg"
  Logical Operator6/1 -> Data Type Conversion9/1
  Gain1/1 -> Bus Creator/2  "VHAL_AccelPedal2Vol_V"
  Logical Operator3/1 -> Data Type Conversion7/1
  Data Type Conversion15/1 -> Bus Creator/16  "VHAL_SeatSW_flg"
  Data Type Conversion4/1 -> Bus Creator/4  "VHAL_CrashInputDuty_pct"
  Data Type Conversion10/1 -> Bus Creator/11  "VHAL_RLDoorSW_flg"
  Logical Operator5/1 -> Data Type Conversion8/1
  Data Type Conversion1/1 -> Gain/1
  VHAL_PsDoorSW_flg/1 -> Logical Operator6/1
  VHAL_AccelPedal1Vol_Raw/1 -> Data Type Conversion1/1
  Data Type Conversion18/1 -> Bus Creator/10  "VHAL_RRDoorSW_flg"
  VHAL_DrDoorSW_flg/1 -> Logical Operator5/1
  Logical Operator11/1 -> Data Type Conversion13/1
  Logical Operator9/1 -> Data Type Conversion2/1
  Logical Operator4/1 -> Data Type Conversion6/1
  VHAL_RLDoorSW_flg/1 -> Logical Operator8/1
  Logical Operator12/1 -> Data Type Conversion14/1
  Data Type Conversion8/1 -> Bus Creator/8  "VHAL_DrDoorSW_flg"
  Gain/1 -> Bus Creator/1  "VHAL_AccelPedal1Vol_V"
  VHAL_HoodSW_flg/1 -> Logical Operator4/1
  Logical Operator10/1 -> Data Type Conversion12/1
  Data Type Conversion14/1 -> Bus Creator/15  "VHAL_TrunkHanSW_flg"
  Data Type Conversion13/1 -> Bus Creator/14  "VHAL_BrakeLampSW_flg"
  Logical Operator7/1 -> Data Type Conversion18/1
  Data Type Conversion17/1 -> Gain1/1
  Logical Operator13/1 -> Data Type Conversion15/1
  Data Type Conversion5/1 -> Bus Creator/5  "VHAL_BrakeSWGPIO_flg"
  Data Type Conversion2/1 -> Bus Creator/12  "VHAL_CentralDoorLockSW_flg"
  VHAL_CentralDoorLockSW_flg/1 -> Logical Operator9/1
  Logical Operator2/1 -> Data Type Conversion5/1
  Data Type Conversion6/1 -> Bus Creator/6  "VHAL_HoodSW_flg"
  Data Type Conversion16/1 -> Bus Creator/17  "VHAL_CrashSignalGPIO_flg"
  Ground4/1 -> Data Type Conversion4/1
  Data Type Conversion3/1 -> Bus Creator/3  "VHAL_CrashInputFreq_Hz"
  VHAL_BrakeLampSW_flg/1 -> Logical Operator11/1
  VHAL_AccelPedal2Vol_Raw/1 -> Data Type Conversion17/1
  VHAL_TailgateSW_flg/1 -> Logical Operator3/1
  Data Type Conversion12/1 -> Bus Creator/13  "VHAL_HazardSW_flg"
  Ground3/1 -> Data Type Conversion3/1
  VHAL_TrunkHanSW_flg/1 -> Logical Operator12/1
  VHAL_RRDoorSW_flg/1 -> Logical Operator7/1
  VHAL_HazardSW_flg/1 -> Logical Operator10/1
  Logical Operator8/1 -> Data Type Conversion10/1
  VHAL_CrashSignalGPIO_flg/1 -> Data Type Conversion16/1
  VHAL_SeatSW_flg/1 -> Logical Operator13/1
  VHAL_BrakeSWGPIO_flg/1 -> Logical Operator2/1
  Bus Creator/1 -> BHAL_GPIO_outputs/1
  Demux/2 -> [VHAL_HWID2_enum]
  Demux/3 -> [VHAL_HWID3_enum]
  Demux/1 -> [VHAL_HWID1_enum]
  Demux/4 -> [VHAL_HWID4_enum]
  u8_HWID_4byte/1 -> Demux/1
  [VHAL_HWID2_enum] -> Data Type Conversion19/1
  [VHAL_HWID3_enum] -> Data Type Conversion20/1
  Data Type Conversion11/1 -> Bus Creator/18  "VHAL_HWID1_enum"
  Data Type Conversion19/1 -> Bus Creator/19  "VHAL_HWID2_enum"
  Data Type Conversion20/1 -> Bus Creator/20  "VHAL_HWID3_enum"
  [VHAL_HWID4_enum] -> Data Type Conversion21/1
  Data Type Conversion21/1 -> Bus Creator/21  "VHAL_HWID4_enum"
  [VHAL_HWID1_enum] -> Data Type Conversion11/1

== system SWC_FDC_type/run_SWC_FDC_RxTx_5ms_sys/Halin_CDD/Halin_IMU ==
  VHAL_IMUOffsetVal_raw : Inport
  VHAL_IMUSixAxisVal_raw : Inport  Port=2
  VHAL_IMUOffsetValSta_flg : Inport  Port=3
  VHAL_IMUSixAxisValSta_flg : Inport  Port=4
  Bus Creator : BusCreator  Inputs=12
  Constant{,1..4} (5 alike) : Constant  Value=0  OutDataTypeStr=int16
  Constant5 : Constant  Value=2000  OutDataTypeStr=int16
  Data Type Conversion{,1..11} (12 alike) : DataTypeConversion  OutDataTypeStr=int16
  Data Type Conversion12 : DataTypeConversion  OutDataTypeStr=boolean
  Data Type Conversion13 : DataTypeConversion  OutDataTypeStr=boolean
  Demux : Demux  Outputs=6
  Demux1 : Demux  Outputs=6
  Switch{,1..11} (12 alike) : Switch  Criteria=u2 ~= 0
  Unit Delay{6..11} (6 alike) : UnitDelay  SampleTime=-1  HasFrameUpgradeWarning=on
  BHAL_IMU_outputs : Outport
  wires:
  Demux1/2 -> Data Type Conversion7/1
  Bus Creator/1 -> BHAL_IMU_outputs/1
  Demux1/3 -> Data Type Conversion8/1
  Demux1/6 -> Data Type Conversion11/1
  Demux/1 -> Data Type Conversion/1
  Demux1/5 -> Data Type Conversion10/1
  Demux/6 -> Data Type Conversion5/1
  Demux/4 -> Data Type Conversion3/1
  Demux/5 -> Data Type Conversion4/1
  Demux1/4 -> Data Type Conversion9/1
  [VHAL_MemOffsetGyroX_raw16] -> Switch/3
  Demux1/1 -> Data Type Conversion6/1
  Demux/2 -> Data Type Conversion1/1
  Demux/3 -> Data Type Conversion2/1
  VHAL_IMUOffsetValSta_flg/1 -> Data Type Conversion12/1
  Switch/1 -> Bus Creator/1  "VHAL_MemOffsetGyroX_raw16"
  [VHAL_IMUOffsetValSta_flg] -> Switch/2
  Switch1/1 -> Bus Creator/2  "VHAL_MemOffsetGyroY_raw16"
  [VHAL_MemOffsetGyroY_raw16] -> Switch1/3
  [VHAL_MemOffsetGyroZ_raw16] -> Switch2/3
  Switch2/1 -> Bus Creator/3  "VHAL_MemOffsetGyroZ_raw16"
  Switch3/1 -> Bus Creator/4  "VHAL_MemOffsetAccX_raw16"
  [VHAL_MemOffsetAccX_raw16] -> Switch3/3
  [VHAL_MemOffsetAccY_raw16] -> Switch4/3
  Switch4/1 -> Bus Creator/5  "VHAL_MemOffsetAccY_raw16"
  Switch5/1 -> Bus Creator/6  "VHAL_MemOffsetAccZ_raw16"
  [VHAL_MemOffsetAccZ_raw16] -> Switch5/3
  [VHAL_SensingGyroX_raw16] -> Switch6/3
  Switch6/1 -> Bus Creator/7, Unit Delay6/1  "VHAL_SensingGyroX_raw16"
  Unit Delay6/1 -> Switch6/1
  Unit Delay7/1 -> Switch7/1
  Switch7/1 -> Bus Creator/8, Unit Delay7/1  "VHAL_SensingGyroY_raw16"
  [VHAL_SensingGyroY_raw16] -> Switch7/3
  [VHAL_SensingGyroZ_raw16] -> Switch8/3
  Switch8/1 -> Bus Creator/9, Unit Delay8/1  "VHAL_SensingGyroZ_raw16"
  Unit Delay8/1 -> Switch8/1
  Unit Delay9/1 -> Switch9/1
  Switch9/1 -> Bus Creator/10, Unit Delay9/1  "VHAL_SensingAccX_raw16"
  [VHAL_SensingAccX_raw16] -> Switch9/3
  [VHAL_SensingAccY_raw16] -> Switch10/3
  Switch10/1 -> Bus Creator/11, Unit Delay10/1  "VHAL_SensingAccY_raw16"
  Unit Delay10/1 -> Switch10/1
  Unit Delay11/1 -> Switch11/1
  Switch11/1 -> Bus Creator/12, Unit Delay11/1  "VHAL_SensingAccZ_raw16"
  [VHAL_SensingAccZ_raw16] -> Switch11/3
  Constant/1 -> Switch/1
  Constant1/1 -> Switch1/1
  [VHAL_IMUOffsetValSta_flg] -> Switch1/2
  Constant2/1 -> Switch2/1
  [VHAL_IMUOffsetValSta_flg] -> Switch2/2
  Constant3/1 -> Switch3/1
  [VHAL_IMUOffsetValSta_flg] -> Switch3/2
  Constant4/1 -> Switch4/1
  [VHAL_IMUOffsetValSta_flg] -> Switch4/2
  Constant5/1 -> Switch5/1
  [VHAL_IMUOffsetValSta_flg] -> Switch5/2
  [VHAL_IMUSixAxisValSta_flg] -> Switch6/2
  [VHAL_IMUSixAxisValSta_flg] -> Switch7/2
  [VHAL_IMUSixAxisValSta_flg] -> Switch8/2
  [VHAL_IMUSixAxisValSta_flg] -> Switch9/2
  [VHAL_IMUSixAxisValSta_flg] -> Switch10/2
  [VHAL_IMUSixAxisValSta_flg] -> Switch11/2
  VHAL_IMUOffsetVal_raw/1 -> Demux/1
  VHAL_IMUSixAxisVal_raw/1 -> Demux1/1
  Data Type Conversion/1 -> [VHAL_MemOffsetAccX_raw16]
  Data Type Conversion1/1 -> [VHAL_MemOffsetAccY_raw16]
  Data Type Conversion2/1 -> [VHAL_MemOffsetAccZ_raw16]
  Data Type Conversion3/1 -> [VHAL_MemOffsetGyroX_raw16]
  Data Type Conversion4/1 -> [VHAL_MemOffsetGyroY_raw16]
  Data Type Conversion5/1 -> [VHAL_MemOffsetGyroZ_raw16]
  Data Type Conversion6/1 -> [VHAL_SensingAccX_raw16]
  Data Type Conversion8/1 -> [VHAL_SensingAccZ_raw16]
  Data Type Conversion7/1 -> [VHAL_SensingAccY_raw16]
  Data Type Conversion10/1 -> [VHAL_SensingGyroY_raw16]
  Data Type Conversion9/1 -> [VHAL_SensingGyroX_raw16]
  Data Type Conversion11/1 -> [VHAL_SensingGyroZ_raw16]
  Data Type Conversion12/1 -> [VHAL_IMUOffsetValSta_flg]  "VHAL_IMUOffsetValSta_flg"
  Data Type Conversion13/1 -> [VHAL_IMUSixAxisValSta_flg]  "VHAL_IMUSixAxisValSta_flg"
  VHAL_IMUSixAxisValSta_flg/1 -> Data Type Conversion13/1
